simulink model "c00012M_harness"  (R2018a)
settings: Solver=FixedStepAuto  StartTime=0.0  StopTime=300  FixedStep=0.1  RelTol=1e-3
undefined symbols (not defined in the file): A1, hmax, PriorityTank, R1, R2, sigbuilder_block
(part 1 of 19)
settings Model: Creator=aarrieta  LastModifiedBy=umarkiegi

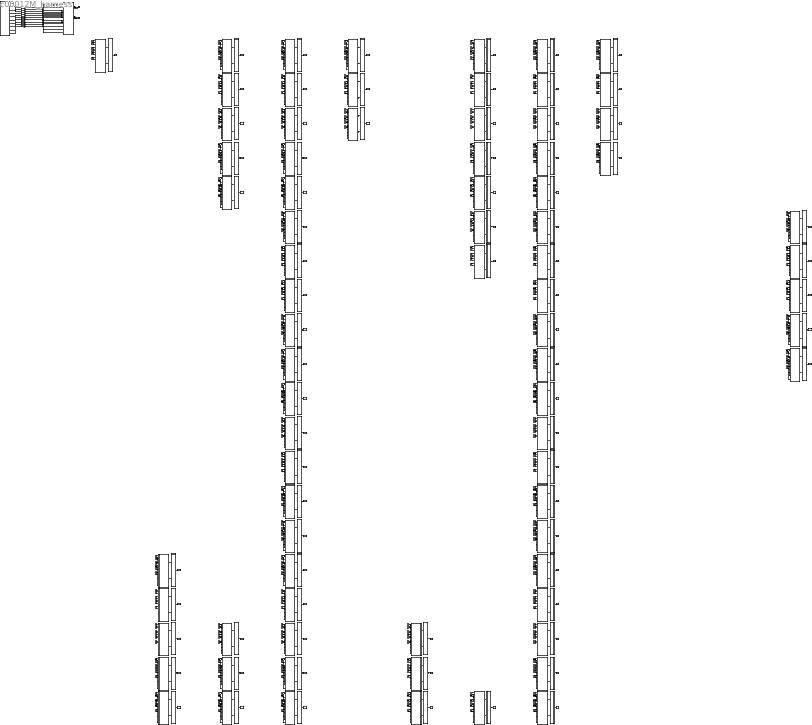
== system c00012M_harness ==
  CPSUT : Subsystem
  Eval : Subsystem
  Eval117 : Subsystem
  Eval118 : Subsystem
  Eval119 : Subsystem
  Eval120 : Subsystem
  Eval121 : Subsystem
  Eval122 : Subsystem
  Eval123 : Subsystem
  Eval124 : Subsystem
  Eval125 : Subsystem
  Eval126 : Subsystem
  Eval139 : Subsystem
  Eval140 : Subsystem
  Eval141 : Subsystem
  Eval142 : Subsystem
  Eval143 : Subsystem
  Eval144 : Subsystem
  Eval145 : Subsystem
  Eval146 : Subsystem
  Eval147 : Subsystem
  Eval148 : Subsystem
  Eval149 : Subsystem
  Eval150 : Subsystem
  Eval151 : Subsystem
  Eval152 : Subsystem
  Eval153 : Subsystem
  Eval154 : Subsystem
  Eval155 : Subsystem
  Eval156 : Subsystem
  Eval157 : Subsystem
  Eval158 : Subsystem
  Eval159 : Subsystem
  Eval160 : Subsystem
  Eval161 : Subsystem
  Eval162 : Subsystem
  Eval163 : Subsystem
  Eval225 : Subsystem
  Eval226 : Subsystem
  Eval227 : Subsystem
  Eval228 : Subsystem
  Eval229 : Subsystem
  Eval35 : Subsystem
  Eval36 : Subsystem
  Eval37 : Subsystem
  Eval38 : Subsystem
  Eval39 : Subsystem
  Eval40 : Subsystem
  Eval41 : Subsystem
  Eval42 : Subsystem
  Eval43 : Subsystem
  Eval44 : Subsystem
  Eval57 : Subsystem
  Eval58 : Subsystem
  Eval59 : Subsystem
  Eval60 : Subsystem
  Eval61 : Subsystem
  Eval62 : Subsystem
  Eval63 : Subsystem
  Eval64 : Subsystem
  Eval65 : Subsystem
  Eval66 : Subsystem
  Eval67 : Subsystem
  Eval68 : Subsystem
  Eval69 : Subsystem
  Eval70 : Subsystem
  Eval71 : Subsystem
  Eval72 : Subsystem
  Eval73 : Subsystem
  Eval74 : Subsystem
  Eval75 : Subsystem
  Eval76 : Subsystem
  Eval77 : Subsystem
  Eval78 : Subsystem
  Eval79 : Subsystem
  Eval80 : Subsystem
  Eval81 : Subsystem
  Eval82 : Subsystem
  Inputs : Subsystem  Tag=STV Subsys  LoadFcn=sigbuilder_block('load');  StartFcn=sigbuilder_block('start');  StopFcn=sigbuilder_block('stop');  ClipboardFcn=sigbuilder_block('clipboard');  mask(Sigbuilder block){tuvar=[0:10]}
      mask init:
      | if ~strcmp(get_param(bdroot(gcb),'SimulationStatus'),'stopped'),tuvar = sigbuilder_block('maskInit'); end
      settings: CopyFcn=sigbuilder_block('copy');  DeleteFcn=sigbuilder_block('delete');  ModelCloseFcn=sigbuilder_block('modelClose');  PreSaveFcn=sigbuilder_block('preSave');  PauseFcn=sigbuilder_block('pause');  ContinueFcn=sigbuilder_block('continue');  NameChangeFcn=sigbuilder_block('namechange');  OpenFcn=sigbuilder_block('open',[276.75 163.5 675.75 486.75 ]);  CloseFcn=sigbuilder_block('close');
      mask Display: plot(0, 0, 100, 100,[2, 2, 32, 32, 2], [68, 8, 8, 68, 68],[32, 2], [38, 38], [32, 19, 2],[53, 60, 44], [32, 17, 17, 2],[16, 16, 31, 31]);txt = getActiveGroup(gcbh);text(2, 100, txt,'verticalAlignment', 'top');
  M001 : Subsystem
  M036 : Subsystem
  M037 : Subsystem
  M038 : Subsystem
  M039 : Subsystem
  M040 : Subsystem
  M041 : Subsystem
  M042 : Subsystem
  M043 : Subsystem
  M044 : Subsystem
  M045 : Subsystem
  M058 : Subsystem
  M059 : Subsystem
  M060 : Subsystem
  M061 : Subsystem
  M062 : Subsystem
  M063 : Subsystem
  M064 : Subsystem
  M065 : Subsystem
  M066 : Subsystem
  M067 : Subsystem
  M068 : Subsystem
  M069 : Subsystem
  M070 : Subsystem
  M071 : Subsystem
  M072 : Subsystem
  M073 : Subsystem
  M074 : Subsystem
  M075 : Subsystem
  M076 : Subsystem
  M077 : Subsystem
  M078 : Subsystem
  M079 : Subsystem
  M080 : Subsystem
  M081 : Subsystem
  M082 : Subsystem
  M083 : Subsystem
  M118 : Subsystem
  M119 : Subsystem
  M120 : Subsystem
  M121 : Subsystem
  M122 : Subsystem
  M123 : Subsystem
  M124 : Subsystem
  M125 : Subsystem
  M126 : Subsystem
  M127 : Subsystem
  M140 : Subsystem
  M141 : Subsystem
  M142 : Subsystem
  M143 : Subsystem
  M144 : Subsystem
  M145 : Subsystem
  M146 : Subsystem
  M147 : Subsystem
  M148 : Subsystem
  M149 : Subsystem
  M150 : Subsystem
  M151 : Subsystem
  M152 : Subsystem
  M153 : Subsystem
  M154 : Subsystem
  M155 : Subsystem
  M156 : Subsystem
  M157 : Subsystem
  M158 : Subsystem
  M159 : Subsystem
  M160 : Subsystem
  M161 : Subsystem
  M162 : Subsystem
  M163 : Subsystem
  M164 : Subsystem
  M226 : Subsystem
  M227 : Subsystem
  M228 : Subsystem
  M229 : Subsystem
  M230 : Subsystem
  To Workspace : ToWorkspace  VariableName=mutant001  SampleTime=-1
  To Workspace117 : ToWorkspace  VariableName=mutant118  SampleTime=-1
  To Workspace118 : ToWorkspace  VariableName=mutant119  SampleTime=-1
  To Workspace119 : ToWorkspace  VariableName=mutant120  SampleTime=-1
  To Workspace120 : ToWorkspace  VariableName=mutant121  SampleTime=-1
  To Workspace121 : ToWorkspace  VariableName=mutant122  SampleTime=-1
  To Workspace122 : ToWorkspace  VariableName=mutant123  SampleTime=-1
  To Workspace123 : ToWorkspace  VariableName=mutant124  SampleTime=-1
  To Workspace124 : ToWorkspace  VariableName=mutant125  SampleTime=-1
  To Workspace125 : ToWorkspace  VariableName=mutant126  SampleTime=-1
  To Workspace126 : ToWorkspace  VariableName=mutant127  SampleTime=-1
  To Workspace139 : ToWorkspace  VariableName=mutant140  SampleTime=-1
  To Workspace140 : ToWorkspace  VariableName=mutant141  SampleTime=-1
  To Workspace141 : ToWorkspace  VariableName=mutant142  SampleTime=-1
  To Workspace142 : ToWorkspace  VariableName=mutant143  SampleTime=-1
  To Workspace143 : ToWorkspace  VariableName=mutant144  SampleTime=-1
  To Workspace144 : ToWorkspace  VariableName=mutant145  SampleTime=-1
  To Workspace145 : ToWorkspace  VariableName=mutant146  SampleTime=-1
  To Workspace146 : ToWorkspace  VariableName=mutant147  SampleTime=-1
  To Workspace147 : ToWorkspace  VariableName=mutant148  SampleTime=-1
  To Workspace148 : ToWorkspace  VariableName=mutant149  SampleTime=-1
  To Workspace149 : ToWorkspace  VariableName=mutant150  SampleTime=-1
  To Workspace150 : ToWorkspace  VariableName=mutant151  SampleTime=-1
  To Workspace151 : ToWorkspace  VariableName=mutant152  SampleTime=-1
  To Workspace152 : ToWorkspace  VariableName=mutant153  SampleTime=-1
  To Workspace153 : ToWorkspace  VariableName=mutant154  SampleTime=-1
  To Workspace154 : ToWorkspace  VariableName=mutant155  SampleTime=-1
  To Workspace155 : ToWorkspace  VariableName=mutant156  SampleTime=-1
  To Workspace156 : ToWorkspace  VariableName=mutant157  SampleTime=-1
  To Workspace157 : ToWorkspace  VariableName=mutant158  SampleTime=-1
  To Workspace158 : ToWorkspace  VariableName=mutant159  SampleTime=-1
  To Workspace159 : ToWorkspace  VariableName=mutant160  SampleTime=-1
  To Workspace160 : ToWorkspace  VariableName=mutant161  SampleTime=-1
  To Workspace161 : ToWorkspace  VariableName=mutant162  SampleTime=-1
  To Workspace162 : ToWorkspace  VariableName=mutant163  SampleTime=-1
  To Workspace163 : ToWorkspace  VariableName=mutant164  SampleTime=-1
  To Workspace225 : ToWorkspace  VariableName=mutant226  SampleTime=-1
  To Workspace226 : ToWorkspace  VariableName=mutant227  SampleTime=-1
  To Workspace227 : ToWorkspace  VariableName=mutant228  SampleTime=-1
  To Workspace228 : ToWorkspace  VariableName=mutant229  SampleTime=-1
  To Workspace229 : ToWorkspace  VariableName=mutant230  SampleTime=-1
  To Workspace35 : ToWorkspace  VariableName=mutant036  SampleTime=-1
  To Workspace36 : ToWorkspace  VariableName=mutant037  SampleTime=-1
  To Workspace37 : ToWorkspace  VariableName=mutant038  SampleTime=-1
  To Workspace38 : ToWorkspace  VariableName=mutant039  SampleTime=-1
  To Workspace39 : ToWorkspace  VariableName=mutant040  SampleTime=-1
  To Workspace40 : ToWorkspace  VariableName=mutant041  SampleTime=-1
  To Workspace41 : ToWorkspace  VariableName=mutant042  SampleTime=-1
  To Workspace42 : ToWorkspace  VariableName=mutant043  SampleTime=-1
  To Workspace43 : ToWorkspace  VariableName=mutant044  SampleTime=-1
  To Workspace44 : ToWorkspace  VariableName=mutant045  SampleTime=-1
  To Workspace57 : ToWorkspace  VariableName=mutant058  SampleTime=-1
  To Workspace58 : ToWorkspace  VariableName=mutant059  SampleTime=-1
  To Workspace59 : ToWorkspace  VariableName=mutant060  SampleTime=-1
  To Workspace60 : ToWorkspace  VariableName=mutant061  SampleTime=-1
  To Workspace61 : ToWorkspace  VariableName=mutant062  SampleTime=-1
  To Workspace62 : ToWorkspace  VariableName=mutant063  SampleTime=-1
  To Workspace63 : ToWorkspace  VariableName=mutant064  SampleTime=-1
  To Workspace64 : ToWorkspace  VariableName=mutant065  SampleTime=-1
  To Workspace65 : ToWorkspace  VariableName=mutant066  SampleTime=-1
  To Workspace66 : ToWorkspace  VariableName=mutant067  SampleTime=-1
  To Workspace67 : ToWorkspace  VariableName=mutant068  SampleTime=-1
  To Workspace68 : ToWorkspace  VariableName=mutant069  SampleTime=-1
  To Workspace69 : ToWorkspace  VariableName=mutant070  SampleTime=-1
  To Workspace70 : ToWorkspace  VariableName=mutant071  SampleTime=-1
  To Workspace71 : ToWorkspace  VariableName=mutant072  SampleTime=-1
  To Workspace72 : ToWorkspace  VariableName=mutant073  SampleTime=-1
  To Workspace73 : ToWorkspace  VariableName=mutant074  SampleTime=-1
  To Workspace74 : ToWorkspace  VariableName=mutant075  SampleTime=-1
  To Workspace75 : ToWorkspace  VariableName=mutant076  SampleTime=-1
  To Workspace76 : ToWorkspace  VariableName=mutant077  SampleTime=-1
  To Workspace77 : ToWorkspace  VariableName=mutant078  SampleTime=-1
  To Workspace78 : ToWorkspace  VariableName=mutant079  SampleTime=-1
  To Workspace79 : ToWorkspace  VariableName=mutant080  SampleTime=-1
  To Workspace80 : ToWorkspace  VariableName=mutant081  SampleTime=-1
  To Workspace81 : ToWorkspace  VariableName=mutant082  SampleTime=-1
  To Workspace82 : ToWorkspace  VariableName=mutant083  SampleTime=-1
  dtc_CT1 : DataTypeConversion
  dtc_CT2 : DataTypeConversion
  dtc_E1 : DataTypeConversion
  dtc_E2 : DataTypeConversion
  dtc_EB1 : DataTypeConversion
  dtc_EB2 : DataTypeConversion
  dtc_F1 : DataTypeConversion
  dtc_F2 : DataTypeConversion
  dtc_T1 : DataTypeConversion
  dtc_T2 : DataTypeConversion
  LL1 : Outport
  LL2 : Outport  Port=2
  tag scope: out1=global, out2=global
  wires:
  CPSUT/1(LL1) -> [out1], LL1/1
  CPSUT/2(LL2) -> [out2], LL2/1
  [in1] -> M001/1(CT1)
  [in2] -> M001/2(F1)
  [in3] -> M001/3(E1)
  [in5] -> M001/4(T1)
  [in6] -> M001/5(EB1)
  [in7] -> M001/6(CT2)
  [in8] -> M001/7(F2)
  [in9] -> M001/8(E2)
  [in11] -> M001/9(T2)
  [in12] -> M001/10(EB2)
  Eval/1(Out1) -> To Workspace/1
  M001/1(LL1) -> Eval/1(In1)
  M001/2(LL2) -> Eval/2(In2)
  [in1] -> M036/1(CT1)
  [in2] -> M036/2(F1)
  [in3] -> M036/3(E1)
  [in5] -> M036/4(T1)
  [in6] -> M036/5(EB1)
  [in7] -> M036/6(CT2)
  [in8] -> M036/7(F2)
  [in9] -> M036/8(E2)
  [in11] -> M036/9(T2)
  [in12] -> M036/10(EB2)
  M036/1(LL1) -> Eval35/1(In1)
  M036/2(LL2) -> Eval35/2(In2)
  Eval35/1(Out1) -> To Workspace35/1
  [in1] -> M037/1(CT1)
  [in2] -> M037/2(F1)
  [in3] -> M037/3(E1)
  [in5] -> M037/4(T1)
  [in6] -> M037/5(EB1)
  [in7] -> M037/6(CT2)
  [in8] -> M037/7(F2)
  [in9] -> M037/8(E2)
  [in11] -> M037/9(T2)
  [in12] -> M037/10(EB2)
  M037/1(LL1) -> Eval36/1(In1)
  M037/2(LL2) -> Eval36/2(In2)
  Eval36/1(Out1) -> To Workspace36/1
  [in1] -> M038/1(CT1)
  [in2] -> M038/2(F1)
  [in3] -> M038/3(E1)
  [in5] -> M038/4(T1)
  [in6] -> M038/5(EB1)
  [in7] -> M038/6(CT2)
  [in8] -> M038/7(F2)
  [in9] -> M038/8(E2)
  [in11] -> M038/9(T2)
  [in12] -> M038/10(EB2)
  M038/1(LL1) -> Eval37/1(In1)
  M038/2(LL2) -> Eval37/2(In2)
  Eval37/1(Out1) -> To Workspace37/1
  [in1] -> M039/1(CT1)
  [in2] -> M039/2(F1)
  [in3] -> M039/3(E1)
  [in5] -> M039/4(T1)
  [in6] -> M039/5(EB1)
  [in7] -> M039/6(CT2)
  [in8] -> M039/7(F2)
  [in9] -> M039/8(E2)
  [in11] -> M039/9(T2)
  [in12] -> M039/10(EB2)
  M039/1(LL1) -> Eval38/1(In1)
  M039/2(LL2) -> Eval38/2(In2)
  Eval38/1(Out1) -> To Workspace38/1
  [in1] -> M040/1(CT1)
  [in2] -> M040/2(F1)
  [in3] -> M040/3(E1)
  [in5] -> M040/4(T1)
  [in6] -> M040/5(EB1)
  [in7] -> M040/6(CT2)
  [in8] -> M040/7(F2)
  [in9] -> M040/8(E2)
  [in11] -> M040/9(T2)
  [in12] -> M040/10(EB2)
  M040/1(LL1) -> Eval39/1(In1)
  M040/2(LL2) -> Eval39/2(In2)
  Eval39/1(Out1) -> To Workspace39/1
  [in1] -> M041/1(CT1)
  [in2] -> M041/2(F1)
  [in3] -> M041/3(E1)
  [in5] -> M041/4(T1)
  [in6] -> M041/5(EB1)
  [in7] -> M041/6(CT2)
  [in8] -> M041/7(F2)
  [in9] -> M041/8(E2)
  [in11] -> M041/9(T2)
  [in12] -> M041/10(EB2)
  M041/1(LL1) -> Eval40/1(In1)
  M041/2(LL2) -> Eval40/2(In2)
  Eval40/1(Out1) -> To Workspace40/1
  [in1] -> M042/1(CT1)
  [in2] -> M042/2(F1)
  [in3] -> M042/3(E1)
  [in5] -> M042/4(T1)
  [in6] -> M042/5(EB1)
  [in7] -> M042/6(CT2)
  [in8] -> M042/7(F2)
  [in9] -> M042/8(E2)
  [in11] -> M042/9(T2)
  [in12] -> M042/10(EB2)
  M042/1(LL1) -> Eval41/1(In1)
  M042/2(LL2) -> Eval41/2(In2)
  Eval41/1(Out1) -> To Workspace41/1
  [in1] -> M043/1(CT1)
  [in2] -> M043/2(F1)
  [in3] -> M043/3(E1)
  [in5] -> M043/4(T1)
  [in6] -> M043/5(EB1)
  [in7] -> M043/6(CT2)
  [in8] -> M043/7(F2)
  [in9] -> M043/8(E2)
  [in11] -> M043/9(T2)
  [in12] -> M043/10(EB2)
  M043/1(LL1) -> Eval42/1(In1)
  M043/2(LL2) -> Eval42/2(In2)
  Eval42/1(Out1) -> To Workspace42/1
  [in1] -> M044/1(CT1)
  [in2] -> M044/2(F1)
  [in3] -> M044/3(E1)
  [in5] -> M044/4(T1)
  [in6] -> M044/5(EB1)
  [in7] -> M044/6(CT2)
  [in8] -> M044/7(F2)
  [in9] -> M044/8(E2)
  [in11] -> M044/9(T2)
  [in12] -> M044/10(EB2)
  M044/1(LL1) -> Eval43/1(In1)
  M044/2(LL2) -> Eval43/2(In2)
  Eval43/1(Out1) -> To Workspace43/1
  [in1] -> M045/1(CT1)
  [in2] -> M045/2(F1)
  [in3] -> M045/3(E1)
  [in5] -> M045/4(T1)
  [in6] -> M045/5(EB1)
  [in7] -> M045/6(CT2)
  [in8] -> M045/7(F2)
  [in9] -> M045/8(E2)
  [in11] -> M045/9(T2)
  [in12] -> M045/10(EB2)
  M045/1(LL1) -> Eval44/1(In1)
  M045/2(LL2) -> Eval44/2(In2)
  Eval44/1(Out1) -> To Workspace44/1
  [in1] -> M058/1(CT1)
  [in2] -> M058/2(F1)
  [in3] -> M058/3(E1)
  [in5] -> M058/4(T1)
  [in6] -> M058/5(EB1)
  [in7] -> M058/6(CT2)
  [in8] -> M058/7(F2)
  [in9] -> M058/8(E2)
  [in11] -> M058/9(T2)
  [in12] -> M058/10(EB2)
  M058/1(LL1) -> Eval57/1(In1)
  M058/2(LL2) -> Eval57/2(In2)
  Eval57/1(Out1) -> To Workspace57/1
  [in1] -> M059/1(CT1)
  [in2] -> M059/2(F1)
  [in3] -> M059/3(E1)
  [in5] -> M059/4(T1)
  [in6] -> M059/5(EB1)
  [in7] -> M059/6(CT2)
  [in8] -> M059/7(F2)
  [in9] -> M059/8(E2)
  [in11] -> M059/9(T2)
  [in12] -> M059/10(EB2)
  M059/1(LL1) -> Eval58/1(In1)
  M059/2(LL2) -> Eval58/2(In2)
  Eval58/1(Out1) -> To Workspace58/1
  [in1] -> M060/1(CT1)
  [in2] -> M060/2(F1)
  [in3] -> M060/3(E1)
  [in5] -> M060/4(T1)
  [in6] -> M060/5(EB1)
  [in7] -> M060/6(CT2)
  [in8] -> M060/7(F2)
  [in9] -> M060/8(E2)
  [in11] -> M060/9(T2)
  [in12] -> M060/10(EB2)
  M060/1(LL1) -> Eval59/1(In1)
  M060/2(LL2) -> Eval59/2(In2)
  Eval59/1(Out1) -> To Workspace59/1
  [in1] -> M061/1(CT1)
  [in2] -> M061/2(F1)
  [in3] -> M061/3(E1)
  [in5] -> M061/4(T1)
  [in6] -> M061/5(EB1)
  [in7] -> M061/6(CT2)
  [in8] -> M061/7(F2)
  [in9] -> M061/8(E2)
  [in11] -> M061/9(T2)
  [in12] -> M061/10(EB2)
  M061/1(LL1) -> Eval60/1(In1)
  M061/2(LL2) -> Eval60/2(In2)
  Eval60/1(Out1) -> To Workspace60/1
  [in1] -> M062/1(CT1)
  [in2] -> M062/2(F1)
  [in3] -> M062/3(E1)
  [in5] -> M062/4(T1)
  [in6] -> M062/5(EB1)
  [in7] -> M062/6(CT2)
  [in8] -> M062/7(F2)
  [in9] -> M062/8(E2)
  [in11] -> M062/9(T2)
  [in12] -> M062/10(EB2)
  M062/1(LL1) -> Eval61/1(In1)
  M062/2(LL2) -> Eval61/2(In2)
  Eval61/1(Out1) -> To Workspace61/1
  [in1] -> M063/1(CT1)
  [in2] -> M063/2(F1)
  [in3] -> M063/3(E1)
  [in5] -> M063/4(T1)
  [in6] -> M063/5(EB1)
  [in7] -> M063/6(CT2)
  [in8] -> M063/7(F2)
  [in9] -> M063/8(E2)
  [in11] -> M063/9(T2)
  [in12] -> M063/10(EB2)
  M063/1(LL1) -> Eval62/1(In1)
  M063/2(LL2) -> Eval62/2(In2)
  Eval62/1(Out1) -> To Workspace62/1
  [in1] -> M064/1(CT1)
  [in2] -> M064/2(F1)
  [in3] -> M064/3(E1)
  [in5] -> M064/4(T1)
  [in6] -> M064/5(EB1)
  [in7] -> M064/6(CT2)
  [in8] -> M064/7(F2)
  [in9] -> M064/8(E2)
  [in11] -> M064/9(T2)
  [in12] -> M064/10(EB2)
  M064/1(LL1) -> Eval63/1(In1)
  M064/2(LL2) -> Eval63/2(In2)
  Eval63/1(Out1) -> To Workspace63/1
  [in1] -> M065/1(CT1)
  [in2] -> M065/2(F1)
  [in3] -> M065/3(E1)
  [in5] -> M065/4(T1)
  [in6] -> M065/5(EB1)
  [in7] -> M065/6(CT2)
  [in8] -> M065/7(F2)
  [in9] -> M065/8(E2)
  [in11] -> M065/9(T2)
  [in12] -> M065/10(EB2)
  M065/1(LL1) -> Eval64/1(In1)
  M065/2(LL2) -> Eval64/2(In2)
  Eval64/1(Out1) -> To Workspace64/1
  [in1] -> M066/1(CT1)
  [in2] -> M066/2(F1)
  [in3] -> M066/3(E1)
  [in5] -> M066/4(T1)
  [in6] -> M066/5(EB1)
  [in7] -> M066/6(CT2)
  [in8] -> M066/7(F2)
  [in9] -> M066/8(E2)
  [in11] -> M066/9(T2)
  [in12] -> M066/10(EB2)
  M066/1(LL1) -> Eval65/1(In1)
  M066/2(LL2) -> Eval65/2(In2)
  Eval65/1(Out1) -> To Workspace65/1
  [in1] -> M067/1(CT1)
  [in2] -> M067/2(F1)
  [in3] -> M067/3(E1)
  [in5] -> M067/4(T1)
  [in6] -> M067/5(EB1)
  [in7] -> M067/6(CT2)
  [in8] -> M067/7(F2)
  [in9] -> M067/8(E2)
  [in11] -> M067/9(T2)
  [in12] -> M067/10(EB2)
  M067/1(LL1) -> Eval66/1(In1)
  M067/2(LL2) -> Eval66/2(In2)
  Eval66/1(Out1) -> To Workspace66/1
  [in1] -> M068/1(CT1)
  [in2] -> M068/2(F1)
  [in3] -> M068/3(E1)
  [in5] -> M068/4(T1)
  [in6] -> M068/5(EB1)
  [in7] -> M068/6(CT2)
  [in8] -> M068/7(F2)
  [in9] -> M068/8(E2)
  [in11] -> M068/9(T2)
  [in12] -> M068/10(EB2)
  M068/1(LL1) -> Eval67/1(In1)
  M068/2(LL2) -> Eval67/2(In2)
  Eval67/1(Out1) -> To Workspace67/1
  [in1] -> M069/1(CT1)
  [in2] -> M069/2(F1)
  [in3] -> M069/3(E1)
  [in5] -> M069/4(T1)
  [in6] -> M069/5(EB1)
  [in7] -> M069/6(CT2)
  [in8] -> M069/7(F2)
  [in9] -> M069/8(E2)
  [in11] -> M069/9(T2)
  [in12] -> M069/10(EB2)
  M069/1(LL1) -> Eval68/1(In1)
  M069/2(LL2) -> Eval68/2(In2)
  Eval68/1(Out1) -> To Workspace68/1
  [in1] -> M070/1(CT1)
  [in2] -> M070/2(F1)
  [in3] -> M070/3(E1)
  [in5] -> M070/4(T1)
  [in6] -> M070/5(EB1)
  [in7] -> M070/6(CT2)
  [in8] -> M070/7(F2)
  [in9] -> M070/8(E2)
  [in11] -> M070/9(T2)
  [in12] -> M070/10(EB2)
  M070/1(LL1) -> Eval69/1(In1)
  M070/2(LL2) -> Eval69/2(In2)
  Eval69/1(Out1) -> To Workspace69/1
  [in1] -> M071/1(CT1)
  [in2] -> M071/2(F1)
  [in3] -> M071/3(E1)
  [in5] -> M071/4(T1)
  [in6] -> M071/5(EB1)
  [in7] -> M071/6(CT2)
  [in8] -> M071/7(F2)
  [in9] -> M071/8(E2)
  [in11] -> M071/9(T2)
  [in12] -> M071/10(EB2)
  M071/1(LL1) -> Eval70/1(In1)
  M071/2(LL2) -> Eval70/2(In2)
  Eval70/1(Out1) -> To Workspace70/1
  [in1] -> M072/1(CT1)
  [in2] -> M072/2(F1)
  [in3] -> M072/3(E1)
  [in5] -> M072/4(T1)
  [in6] -> M072/5(EB1)
  [in7] -> M072/6(CT2)
  [in8] -> M072/7(F2)
  [in9] -> M072/8(E2)
  [in11] -> M072/9(T2)
  [in12] -> M072/10(EB2)
  M072/1(LL1) -> Eval71/1(In1)
  M072/2(LL2) -> Eval71/2(In2)
  Eval71/1(Out1) -> To Workspace71/1
  [in1] -> M073/1(CT1)
  [in2] -> M073/2(F1)
  [in3] -> M073/3(E1)
  [in5] -> M073/4(T1)
  [in6] -> M073/5(EB1)
  [in7] -> M073/6(CT2)
  [in8] -> M073/7(F2)
  [in9] -> M073/8(E2)
  [in11] -> M073/9(T2)
  [in12] -> M073/10(EB2)
  M073/1(LL1) -> Eval72/1(In1)
  M073/2(LL2) -> Eval72/2(In2)
  Eval72/1(Out1) -> To Workspace72/1
  [in1] -> M074/1(CT1)
  [in2] -> M074/2(F1)
  [in3] -> M074/3(E1)
  [in5] -> M074/4(T1)
  [in6] -> M074/5(EB1)
  [in7] -> M074/6(CT2)
  [in8] -> M074/7(F2)
  [in9] -> M074/8(E2)
  [in11] -> M074/9(T2)
  [in12] -> M074/10(EB2)
  M074/1(LL1) -> Eval73/1(In1)
  M074/2(LL2) -> Eval73/2(In2)
  Eval73/1(Out1) -> To Workspace73/1
  [in1] -> M075/1(CT1)
  [in2] -> M075/2(F1)
  [in3] -> M075/3(E1)
  [in5] -> M075/4(T1)
  [in6] -> M075/5(EB1)
  [in7] -> M075/6(CT2)
  [in8] -> M075/7(F2)
  [in9] -> M075/8(E2)
  [in11] -> M075/9(T2)
  [in12] -> M075/10(EB2)
  M075/1(LL1) -> Eval74/1(In1)
  M075/2(LL2) -> Eval74/2(In2)
  Eval74/1(Out1) -> To Workspace74/1
  [in1] -> M076/1(CT1)
  [in2] -> M076/2(F1)
  [in3] -> M076/3(E1)
  [in5] -> M076/4(T1)
  [in6] -> M076/5(EB1)
  [in7] -> M076/6(CT2)
  [in8] -> M076/7(F2)
  [in9] -> M076/8(E2)
  [in11] -> M076/9(T2)
  [in12] -> M076/10(EB2)
  M076/1(LL1) -> Eval75/1(In1)
  M076/2(LL2) -> Eval75/2(In2)
  Eval75/1(Out1) -> To Workspace75/1
  [in1] -> M077/1(CT1)
  [in2] -> M077/2(F1)
  [in3] -> M077/3(E1)
  [in5] -> M077/4(T1)
  [in6] -> M077/5(EB1)
  [in7] -> M077/6(CT2)
  [in8] -> M077/7(F2)
  [in9] -> M077/8(E2)
  [in11] -> M077/9(T2)
  [in12] -> M077/10(EB2)
  M077/1(LL1) -> Eval76/1(In1)
  M077/2(LL2) -> Eval76/2(In2)
  Eval76/1(Out1) -> To Workspace76/1
  [in1] -> M078/1(CT1)
  [in2] -> M078/2(F1)
  [in3] -> M078/3(E1)
  [in5] -> M078/4(T1)
  [in6] -> M078/5(EB1)
  [in7] -> M078/6(CT2)
  [in8] -> M078/7(F2)
  [in9] -> M078/8(E2)
  [in11] -> M078/9(T2)
  [in12] -> M078/10(EB2)
  M078/1(LL1) -> Eval77/1(In1)
  M078/2(LL2) -> Eval77/2(In2)
  Eval77/1(Out1) -> To Workspace77/1
  [in1] -> M079/1(CT1)
  [in2] -> M079/2(F1)
  [in3] -> M079/3(E1)
  [in5] -> M079/4(T1)
  [in6] -> M079/5(EB1)
  [in7] -> M079/6(CT2)
  [in8] -> M079/7(F2)
  [in9] -> M079/8(E2)
  [in11] -> M079/9(T2)
  [in12] -> M079/10(EB2)
  M079/1(LL1) -> Eval78/1(In1)
  M079/2(LL2) -> Eval78/2(In2)
  Eval78/1(Out1) -> To Workspace78/1
  [in1] -> M080/1(CT1)
  [in2] -> M080/2(F1)
  [in3] -> M080/3(E1)
  [in5] -> M080/4(T1)
  [in6] -> M080/5(EB1)
  [in7] -> M080/6(CT2)
  [in8] -> M080/7(F2)
  [in9] -> M080/8(E2)
  [in11] -> M080/9(T2)
  [in12] -> M080/10(EB2)
  M080/1(LL1) -> Eval79/1(In1)
  M080/2(LL2) -> Eval79/2(In2)
  Eval79/1(Out1) -> To Workspace79/1
  [in1] -> M081/1(CT1)
  [in2] -> M081/2(F1)
  [in3] -> M081/3(E1)
  [in5] -> M081/4(T1)
  [in6] -> M081/5(EB1)
  [in7] -> M081/6(CT2)
  [in8] -> M081/7(F2)
  [in9] -> M081/8(E2)
  [in11] -> M081/9(T2)
  [in12] -> M081/10(EB2)
  M081/1(LL1) -> Eval80/1(In1)
  M081/2(LL2) -> Eval80/2(In2)
  Eval80/1(Out1) -> To Workspace80/1
  [in1] -> M082/1(CT1)
  [in2] -> M082/2(F1)
  [in3] -> M082/3(E1)
  [in5] -> M082/4(T1)
  [in6] -> M082/5(EB1)
  [in7] -> M082/6(CT2)
  [in8] -> M082/7(F2)
  [in9] -> M082/8(E2)
  [in11] -> M082/9(T2)
  [in12] -> M082/10(EB2)
  M082/1(LL1) -> Eval81/1(In1)
  M082/2(LL2) -> Eval81/2(In2)
  Eval81/1(Out1) -> To Workspace81/1
  [in1] -> M083/1(CT1)
  [in2] -> M083/2(F1)
  [in3] -> M083/3(E1)
  [in5] -> M083/4(T1)
  [in6] -> M083/5(EB1)
  [in7] -> M083/6(CT2)
  [in8] -> M083/7(F2)
  [in9] -> M083/8(E2)
  [in11] -> M083/9(T2)
  [in12] -> M083/10(EB2)
  M083/1(LL1) -> Eval82/1(In1)
  M083/2(LL2) -> Eval82/2(In2)
  Eval82/1(Out1) -> To Workspace82/1
  [in1] -> M118/1(CT1)
  [in2] -> M118/2(F1)
  [in3] -> M118/3(E1)
  [in5] -> M118/4(T1)
  [in6] -> M118/5(EB1)
  [in7] -> M118/6(CT2)
  [in8] -> M118/7(F2)
  [in9] -> M118/8(E2)
  [in11] -> M118/9(T2)
  [in12] -> M118/10(EB2)
  M118/1(LL1) -> Eval117/1(In1)
  M118/2(LL2) -> Eval117/2(In2)
  Eval117/1(Out1) -> To Workspace117/1
  [in1] -> M119/1(CT1)
  [in2] -> M119/2(F1)
  [in3] -> M119/3(E1)
  [in5] -> M119/4(T1)
  [in6] -> M119/5(EB1)
  [in7] -> M119/6(CT2)
  [in8] -> M119/7(F2)
  [in9] -> M119/8(E2)
  [in11] -> M119/9(T2)
  [in12] -> M119/10(EB2)
  M119/1(LL1) -> Eval118/1(In1)
  M119/2(LL2) -> Eval118/2(In2)
  Eval118/1(Out1) -> To Workspace118/1
  [in1] -> M120/1(CT1)
  [in2] -> M120/2(F1)
  [in3] -> M120/3(E1)
  [in5] -> M120/4(T1)
  [in6] -> M120/5(EB1)
  [in7] -> M120/6(CT2)
  [in8] -> M120/7(F2)
  [in9] -> M120/8(E2)
  [in11] -> M120/9(T2)
  [in12] -> M120/10(EB2)
  M120/1(LL1) -> Eval119/1(In1)
  M120/2(LL2) -> Eval119/2(In2)
  Eval119/1(Out1) -> To Workspace119/1
  [in1] -> M121/1(CT1)
  [in2] -> M121/2(F1)
  [in3] -> M121/3(E1)
  [in5] -> M121/4(T1)
  [in6] -> M121/5(EB1)
  [in7] -> M121/6(CT2)
  [in8] -> M121/7(F2)
  [in9] -> M121/8(E2)
  [in11] -> M121/9(T2)
  [in12] -> M121/10(EB2)
  M121/1(LL1) -> Eval120/1(In1)
  M121/2(LL2) -> Eval120/2(In2)
  Eval120/1(Out1) -> To Workspace120/1
  [in1] -> M122/1(CT1)
  [in2] -> M122/2(F1)
  [in3] -> M122/3(E1)
  [in5] -> M122/4(T1)
  [in6] -> M122/5(EB1)
  [in7] -> M122/6(CT2)
  [in8] -> M122/7(F2)
  [in9] -> M122/8(E2)
  [in11] -> M122/9(T2)
  [in12] -> M122/10(EB2)
  M122/1(LL1) -> Eval121/1(In1)
  M122/2(LL2) -> Eval121/2(In2)
  Eval121/1(Out1) -> To Workspace121/1
  [in1] -> M123/1(CT1)
  [in2] -> M123/2(F1)
  [in3] -> M123/3(E1)
  [in5] -> M123/4(T1)
  [in6] -> M123/5(EB1)
  [in7] -> M123/6(CT2)
  [in8] -> M123/7(F2)
  [in9] -> M123/8(E2)
  [in11] -> M123/9(T2)
  [in12] -> M123/10(EB2)
  M123/1(LL1) -> Eval122/1(In1)
  M123/2(LL2) -> Eval122/2(In2)
  Eval122/1(Out1) -> To Workspace122/1
  [in1] -> M124/1(CT1)
  [in2] -> M124/2(F1)
  [in3] -> M124/3(E1)
  [in5] -> M124/4(T1)
  [in6] -> M124/5(EB1)
  [in7] -> M124/6(CT2)
  [in8] -> M124/7(F2)
  [in9] -> M124/8(E2)
  [in11] -> M124/9(T2)
  [in12] -> M124/10(EB2)
  M124/1(LL1) -> Eval123/1(In1)
  M124/2(LL2) -> Eval123/2(In2)
  Eval123/1(Out1) -> To Workspace123/1
  [in1] -> M125/1(CT1)
  [in2] -> M125/2(F1)
  [in3] -> M125/3(E1)
  [in5] -> M125/4(T1)
  [in6] -> M125/5(EB1)
  [in7] -> M125/6(CT2)
  [in8] -> M125/7(F2)
  [in9] -> M125/8(E2)
  [in11] -> M125/9(T2)
  [in12] -> M125/10(EB2)
  M125/1(LL1) -> Eval124/1(In1)
  M125/2(LL2) -> Eval124/2(In2)
  Eval124/1(Out1) -> To Workspace124/1
  [in1] -> M126/1(CT1)
  [in2] -> M126/2(F1)
  [in3] -> M126/3(E1)
  [in5] -> M126/4(T1)
  [in6] -> M126/5(EB1)
  [in7] -> M126/6(CT2)
  [in8] -> M126/7(F2)
  [in9] -> M126/8(E2)
  [in11] -> M126/9(T2)
  [in12] -> M126/10(EB2)
  M126/1(LL1) -> Eval125/1(In1)
  M126/2(LL2) -> Eval125/2(In2)
  Eval125/1(Out1) -> To Workspace125/1
  [in1] -> M127/1(CT1)
  [in2] -> M127/2(F1)
  [in3] -> M127/3(E1)
  [in5] -> M127/4(T1)
  [in6] -> M127/5(EB1)
  [in7] -> M127/6(CT2)
  [in8] -> M127/7(F2)
  [in9] -> M127/8(E2)
  [in11] -> M127/9(T2)
  [in12] -> M127/10(EB2)
  M127/1(LL1) -> Eval126/1(In1)
  M127/2(LL2) -> Eval126/2(In2)
  Eval126/1(Out1) -> To Workspace126/1
  [in1] -> M140/1(CT1)
  [in2] -> M140/2(F1)
  [in3] -> M140/3(E1)
  [in5] -> M140/4(T1)
  [in6] -> M140/5(EB1)
  [in7] -> M140/6(CT2)
  [in8] -> M140/7(F2)
  [in9] -> M140/8(E2)
  [in11] -> M140/9(T2)
  [in12] -> M140/10(EB2)
  M140/1(LL1) -> Eval139/1(In1)
  M140/2(LL2) -> Eval139/2(In2)
  Eval139/1(Out1) -> To Workspace139/1
  [in1] -> M141/1(CT1)
  [in2] -> M141/2(F1)
  [in3] -> M141/3(E1)
  [in5] -> M141/4(T1)
  [in6] -> M141/5(EB1)
  [in7] -> M141/6(CT2)
  [in8] -> M141/7(F2)
  [in9] -> M141/8(E2)
  [in11] -> M141/9(T2)
  [in12] -> M141/10(EB2)
  M141/1(LL1) -> Eval140/1(In1)
  M141/2(LL2) -> Eval140/2(In2)
  Eval140/1(Out1) -> To Workspace140/1
  [in1] -> M142/1(CT1)
  [in2] -> M142/2(F1)
  [in3] -> M142/3(E1)
  [in5] -> M142/4(T1)
  [in6] -> M142/5(EB1)
  [in7] -> M142/6(CT2)
  [in8] -> M142/7(F2)
  [in9] -> M142/8(E2)
  [in11] -> M142/9(T2)
  [in12] -> M142/10(EB2)
  M142/1(LL1) -> Eval141/1(In1)
  M142/2(LL2) -> Eval141/2(In2)
  Eval141/1(Out1) -> To Workspace141/1
  [in1] -> M143/1(CT1)
  [in2] -> M143/2(F1)
  [in3] -> M143/3(E1)
  [in5] -> M143/4(T1)
  [in6] -> M143/5(EB1)
  [in7] -> M143/6(CT2)
  [in8] -> M143/7(F2)
  [in9] -> M143/8(E2)
  [in11] -> M143/9(T2)
  [in12] -> M143/10(EB2)
  M143/1(LL1) -> Eval142/1(In1)
  M143/2(LL2) -> Eval142/2(In2)
  Eval142/1(Out1) -> To Workspace142/1
  [in1] -> M144/1(CT1)
  [in2] -> M144/2(F1)
  [in3] -> M144/3(E1)
  [in5] -> M144/4(T1)
  [in6] -> M144/5(EB1)
  [in7] -> M144/6(CT2)
  [in8] -> M144/7(F2)
  [in9] -> M144/8(E2)
  [in11] -> M144/9(T2)
  [in12] -> M144/10(EB2)
  M144/1(LL1) -> Eval143/1(In1)
  M144/2(LL2) -> Eval143/2(In2)
  Eval143/1(Out1) -> To Workspace143/1
  [in1] -> M145/1(CT1)
  [in2] -> M145/2(F1)
  [in3] -> M145/3(E1)
  [in5] -> M145/4(T1)
  [in6] -> M145/5(EB1)
  [in7] -> M145/6(CT2)
  [in8] -> M145/7(F2)
  [in9] -> M145/8(E2)
  [in11] -> M145/9(T2)
  [in12] -> M145/10(EB2)
  M145/1(LL1) -> Eval144/1(In1)
  M145/2(LL2) -> Eval144/2(In2)
  Eval144/1(Out1) -> To Workspace144/1
  [in1] -> M146/1(CT1)
  [in2] -> M146/2(F1)
  [in3] -> M146/3(E1)
  [in5] -> M146/4(T1)
  [in6] -> M146/5(EB1)
  [in7] -> M146/6(CT2)
  [in8] -> M146/7(F2)
  [in9] -> M146/8(E2)
  [in11] -> M146/9(T2)
  [in12] -> M146/10(EB2)
  M146/1(LL1) -> Eval145/1(In1)
  M146/2(LL2) -> Eval145/2(In2)
  Eval145/1(Out1) -> To Workspace145/1
  [in1] -> M147/1(CT1)
  [in2] -> M147/2(F1)
  [in3] -> M147/3(E1)
  [in5] -> M147/4(T1)
  [in6] -> M147/5(EB1)
  [in7] -> M147/6(CT2)
  [in8] -> M147/7(F2)
  [in9] -> M147/8(E2)
  [in11] -> M147/9(T2)
  [in12] -> M147/10(EB2)
  M147/1(LL1) -> Eval146/1(In1)
  M147/2(LL2) -> Eval146/2(In2)
  Eval146/1(Out1) -> To Workspace146/1
  [in1] -> M148/1(CT1)
  [in2] -> M148/2(F1)
  [in3] -> M148/3(E1)
  [in5] -> M148/4(T1)
  [in6] -> M148/5(EB1)
  [in7] -> M148/6(CT2)
  [in8] -> M148/7(F2)
  [in9] -> M148/8(E2)
  [in11] -> M148/9(T2)
  [in12] -> M148/10(EB2)
  M148/1(LL1) -> Eval147/1(In1)
  M148/2(LL2) -> Eval147/2(In2)
  Eval147/1(Out1) -> To Workspace147/1
  [in1] -> M149/1(CT1)
  [in2] -> M149/2(F1)
  [in3] -> M149/3(E1)
  [in5] -> M149/4(T1)
  [in6] -> M149/5(EB1)
  [in7] -> M149/6(CT2)
  [in8] -> M149/7(F2)
  [in9] -> M149/8(E2)
  [in11] -> M149/9(T2)
  [in12] -> M149/10(EB2)
  M149/1(LL1) -> Eval148/1(In1)
  M149/2(LL2) -> Eval148/2(In2)
  Eval148/1(Out1) -> To Workspace148/1
  [in1] -> M150/1(CT1)
  [in2] -> M150/2(F1)
  [in3] -> M150/3(E1)
  [in5] -> M150/4(T1)
  [in6] -> M150/5(EB1)
  [in7] -> M150/6(CT2)
  [in8] -> M150/7(F2)
  [in9] -> M150/8(E2)
  [in11] -> M150/9(T2)
  [in12] -> M150/10(EB2)
  M150/1(LL1) -> Eval149/1(In1)
  M150/2(LL2) -> Eval149/2(In2)
  Eval149/1(Out1) -> To Workspace149/1
  [in1] -> M151/1(CT1)
  [in2] -> M151/2(F1)
  [in3] -> M151/3(E1)
  [in5] -> M151/4(T1)
  [in6] -> M151/5(EB1)
  [in7] -> M151/6(CT2)
  [in8] -> M151/7(F2)
  [in9] -> M151/8(E2)
  [in11] -> M151/9(T2)
  [in12] -> M151/10(EB2)
  M151/1(LL1) -> Eval150/1(In1)
  M151/2(LL2) -> Eval150/2(In2)
  Eval150/1(Out1) -> To Workspace150/1
  [in1] -> M152/1(CT1)
  [in2] -> M152/2(F1)
  [in3] -> M152/3(E1)
  [in5] -> M152/4(T1)
  [in6] -> M152/5(EB1)
  [in7] -> M152/6(CT2)
  [in8] -> M152/7(F2)
  [in9] -> M152/8(E2)
  [in11] -> M152/9(T2)
  [in12] -> M152/10(EB2)
  M152/1(LL1) -> Eval151/1(In1)
  M152/2(LL2) -> Eval151/2(In2)
  Eval151/1(Out1) -> To Workspace151/1
  [in1] -> M153/1(CT1)
  [in2] -> M153/2(F1)
  [in3] -> M153/3(E1)
  [in5] -> M153/4(T1)
  [in6] -> M153/5(EB1)
  [in7] -> M153/6(CT2)
  [in8] -> M153/7(F2)
  [in9] -> M153/8(E2)
  [in11] -> M153/9(T2)
  [in12] -> M153/10(EB2)
  M153/1(LL1) -> Eval152/1(In1)
  M153/2(LL2) -> Eval152/2(In2)
  Eval152/1(Out1) -> To Workspace152/1
  [in1] -> M154/1(CT1)
  [in2] -> M154/2(F1)
  [in3] -> M154/3(E1)
  [in5] -> M154/4(T1)
  [in6] -> M154/5(EB1)
  [in7] -> M154/6(CT2)
  [in8] -> M154/7(F2)
  [in9] -> M154/8(E2)
  [in11] -> M154/9(T2)
  [in12] -> M154/10(EB2)
  M154/1(LL1) -> Eval153/1(In1)
  M154/2(LL2) -> Eval153/2(In2)
  Eval153/1(Out1) -> To Workspace153/1
  [in1] -> M155/1(CT1)
  [in2] -> M155/2(F1)
  [in3] -> M155/3(E1)
  [in5] -> M155/4(T1)
  [in6] -> M155/5(EB1)
  [in7] -> M155/6(CT2)
  [in8] -> M155/7(F2)
  [in9] -> M155/8(E2)
  [in11] -> M155/9(T2)
  [in12] -> M155/10(EB2)
  M155/1(LL1) -> Eval154/1(In1)
  M155/2(LL2) -> Eval154/2(In2)
  Eval154/1(Out1) -> To Workspace154/1
  [in1] -> M156/1(CT1)
  [in2] -> M156/2(F1)
  [in3] -> M156/3(E1)
  [in5] -> M156/4(T1)
  [in6] -> M156/5(EB1)
  [in7] -> M156/6(CT2)
  [in8] -> M156/7(F2)
  [in9] -> M156/8(E2)
  [in11] -> M156/9(T2)
  [in12] -> M156/10(EB2)
  M156/1(LL1) -> Eval155/1(In1)
  M156/2(LL2) -> Eval155/2(In2)
  Eval155/1(Out1) -> To Workspace155/1
  [in1] -> M157/1(CT1)
  [in2] -> M157/2(F1)
  [in3] -> M157/3(E1)
  [in5] -> M157/4(T1)
  [in6] -> M157/5(EB1)
  [in7] -> M157/6(CT2)
  [in8] -> M157/7(F2)
  [in9] -> M157/8(E2)
  [in11] -> M157/9(T2)
  [in12] -> M157/10(EB2)
  M157/1(LL1) -> Eval156/1(In1)
  M157/2(LL2) -> Eval156/2(In2)
  Eval156/1(Out1) -> To Workspace156/1
  [in1] -> M158/1(CT1)
  [in2] -> M158/2(F1)
  [in3] -> M158/3(E1)
  [in5] -> M158/4(T1)
  [in6] -> M158/5(EB1)
  [in7] -> M158/6(CT2)
  [in8] -> M158/7(F2)
  [in9] -> M158/8(E2)
  [in11] -> M158/9(T2)
  [in12] -> M158/10(EB2)
  M158/1(LL1) -> Eval157/1(In1)
  M158/2(LL2) -> Eval157/2(In2)
  Eval157/1(Out1) -> To Workspace157/1
  [in1] -> M159/1(CT1)
  [in2] -> M159/2(F1)
  [in3] -> M159/3(E1)
  [in5] -> M159/4(T1)
  [in6] -> M159/5(EB1)
  [in7] -> M159/6(CT2)
  [in8] -> M159/7(F2)
  [in9] -> M159/8(E2)
  [in11] -> M159/9(T2)
  [in12] -> M159/10(EB2)
  M159/1(LL1) -> Eval158/1(In1)
  M159/2(LL2) -> Eval158/2(In2)
  Eval158/1(Out1) -> To Workspace158/1
  [in1] -> M160/1(CT1)
  [in2] -> M160/2(F1)
  [in3] -> M160/3(E1)
  [in5] -> M160/4(T1)
  [in6] -> M160/5(EB1)
  [in7] -> M160/6(CT2)
  [in8] -> M160/7(F2)
  [in9] -> M160/8(E2)
  [in11] -> M160/9(T2)
  [in12] -> M160/10(EB2)
  M160/1(LL1) -> Eval159/1(In1)
  M160/2(LL2) -> Eval159/2(In2)
  Eval159/1(Out1) -> To Workspace159/1
  [in1] -> M161/1(CT1)
  [in2] -> M161/2(F1)
  [in3] -> M161/3(E1)
  [in5] -> M161/4(T1)
  [in6] -> M161/5(EB1)
  [in7] -> M161/6(CT2)
  [in8] -> M161/7(F2)
  [in9] -> M161/8(E2)
  [in11] -> M161/9(T2)
  [in12] -> M161/10(EB2)
  M161/1(LL1) -> Eval160/1(In1)
  M161/2(LL2) -> Eval160/2(In2)
  Eval160/1(Out1) -> To Workspace160/1
  [in1] -> M162/1(CT1)
  [in2] -> M162/2(F1)
  [in3] -> M162/3(E1)
  [in5] -> M162/4(T1)
  [in6] -> M162/5(EB1)
  [in7] -> M162/6(CT2)
  [in8] -> M162/7(F2)
  [in9] -> M162/8(E2)
  [in11] -> M162/9(T2)
  [in12] -> M162/10(EB2)
  M162/1(LL1) -> Eval161/1(In1)
  M162/2(LL2) -> Eval161/2(In2)
  Eval161/1(Out1) -> To Workspace161/1
  [in1] -> M163/1(CT1)
  [in2] -> M163/2(F1)
  [in3] -> M163/3(E1)
  [in5] -> M163/4(T1)
  [in6] -> M163/5(EB1)
  [in7] -> M163/6(CT2)
  [in8] -> M163/7(F2)
  [in9] -> M163/8(E2)
  [in11] -> M163/9(T2)
  [in12] -> M163/10(EB2)
  M163/1(LL1) -> Eval162/1(In1)
  M163/2(LL2) -> Eval162/2(In2)
  Eval162/1(Out1) -> To Workspace162/1
  [in1] -> M164/1(CT1)
  [in2] -> M164/2(F1)
  [in3] -> M164/3(E1)
  [in5] -> M164/4(T1)
  [in6] -> M164/5(EB1)
  [in7] -> M164/6(CT2)
  [in8] -> M164/7(F2)
  [in9] -> M164/8(E2)
  [in11] -> M164/9(T2)
  [in12] -> M164/10(EB2)
  M164/1(LL1) -> Eval163/1(In1)
  M164/2(LL2) -> Eval163/2(In2)
  Eval163/1(Out1) -> To Workspace163/1
  [in1] -> M226/1(CT1)
  [in2] -> M226/2(F1)
  [in3] -> M226/3(E1)
  [in5] -> M226/4(T1)
  [in6] -> M226/5(EB1)
  [in7] -> M226/6(CT2)
  [in8] -> M226/7(F2)
  [in9] -> M226/8(E2)
  [in11] -> M226/9(T2)
  [in12] -> M226/10(EB2)
  M226/1(LL1) -> Eval225/1(In1)
  M226/2(LL2) -> Eval225/2(In2)
  Eval225/1(Out1) -> To Workspace225/1
  [in1] -> M227/1(CT1)
  [in2] -> M227/2(F1)
  [in3] -> M227/3(E1)
  [in5] -> M227/4(T1)
  [in6] -> M227/5(EB1)
  [in7] -> M227/6(CT2)
  [in8] -> M227/7(F2)
  [in9] -> M227/8(E2)
  [in11] -> M227/9(T2)
  [in12] -> M227/10(EB2)
  M227/1(LL1) -> Eval226/1(In1)
  M227/2(LL2) -> Eval226/2(In2)
  Eval226/1(Out1) -> To Workspace226/1
  [in1] -> M228/1(CT1)
  [in2] -> M228/2(F1)
  [in3] -> M228/3(E1)
  [in5] -> M228/4(T1)
  [in6] -> M228/5(EB1)
  [in7] -> M228/6(CT2)
  [in8] -> M228/7(F2)
  [in9] -> M228/8(E2)
  [in11] -> M228/9(T2)
  [in12] -> M228/10(EB2)
  M228/1(LL1) -> Eval227/1(In1)
  M228/2(LL2) -> Eval227/2(In2)
  Eval227/1(Out1) -> To Workspace227/1
  [in1] -> M229/1(CT1)
  [in2] -> M229/2(F1)
  [in3] -> M229/3(E1)
  [in5] -> M229/4(T1)
  [in6] -> M229/5(EB1)
  [in7] -> M229/6(CT2)
  [in8] -> M229/7(F2)
  [in9] -> M229/8(E2)
  [in11] -> M229/9(T2)
  [in12] -> M229/10(EB2)
  M229/1(LL1) -> Eval228/1(In1)
  M229/2(LL2) -> Eval228/2(In2)
  Eval228/1(Out1) -> To Workspace228/1
  [in1] -> M230/1(CT1)
  [in2] -> M230/2(F1)
  [in3] -> M230/3(E1)
  [in5] -> M230/4(T1)
  [in6] -> M230/5(EB1)
  [in7] -> M230/6(CT2)
  [in8] -> M230/7(F2)
  [in9] -> M230/8(E2)
  [in11] -> M230/9(T2)
  [in12] -> M230/10(EB2)
  M230/1(LL1) -> Eval229/1(In1)
  M230/2(LL2) -> Eval229/2(In2)
  Eval229/1(Out1) -> To Workspace229/1
  Inputs/1(CT1) -> dtc_CT1/1
  dtc_CT1/1 -> CPSUT/1(CT1), [in1]
  Inputs/2(F1) -> dtc_F1/1
  dtc_F1/1 -> CPSUT/2(F1), [in2]
  Inputs/3(E1) -> dtc_E1/1
  dtc_E1/1 -> CPSUT/3(E1), [in3]
  Inputs/4(T1) -> dtc_T1/1
  dtc_T1/1 -> CPSUT/4(T1), [in5]
  Inputs/5(EB1) -> dtc_EB1/1
  dtc_EB1/1 -> CPSUT/5(EB1), [in6]
  Inputs/6(CT2) -> dtc_CT2/1
  dtc_CT2/1 -> CPSUT/6(CT2), [in7]
  Inputs/7(F2) -> dtc_F2/1
  dtc_F2/1 -> CPSUT/7(F2), [in8]
  Inputs/8(E2) -> dtc_E2/1
  dtc_E2/1 -> CPSUT/8(E2), [in9]
  Inputs/9(T2) -> dtc_T2/1
  dtc_T2/1 -> CPSUT/9(T2), [in11]
  Inputs/10(EB2) -> dtc_EB2/1
  dtc_EB2/1 -> CPSUT/10(EB2), [in12]

== system c00012M_harness/CPSUT ==
  note: VALUES
      | ---------------------------------
      | ControlType = 1 | 2 | 3
      | FillTank = 0 | 1
      | EmptyTank = 0 | 1
      | ManualReference between 0 and 1
      | Tempreature between 0 and 100
      | EmergencyButton = 0 | 1
      | LiquidLevel between 0 and 1 (hmax)
  note: Inputs For Tank2
  note: NAMES
      | --------------------------------------------
      | CT1 = ControlType Tank 1
      | F1 = Fill Tank 1
      | E1 = Empty Tank 1
      | MR1 = Manual Reference Tank1
      | T1 = Temperature Tank 1
      | EB1 = Emergency Button Tank 1
      | LL1 = Liquid Level 1
  note: Inputs For Tank3
  note: Inputs For Tank1
  CT1 : Inport
  F1 : Inport  Port=2
  E1 : Inport  Port=3
  T1 : Inport  Port=4
  EB1 : Inport  Port=5
  CT2 : Inport  Port=6
  F2 : Inport  Port=7
  E2 : Inport  Port=8
  T2 : Inport  Port=9
  EB2 : Inport  Port=10
  Tank1 : Subsystem
  Tank2 : Subsystem
  LL1 : Outport
  LL2 : Outport  Port=2
  wires:
  EB1/1 -> Tank1/5(EB1)
  Tank2/1(LL2) -> LL2/1, Tank1/6(LL2)
  EB2/1 -> Tank2/5(EB2)
  CT2/1 -> Tank2/1(CT2)
  T1/1 -> Tank1/4(T1)
  Tank1/1(LL1) -> LL1/1, Tank2/6(LL1)
  F2/1 -> Tank2/2(F2)
  E2/1 -> Tank2/3(E2)
  F1/1 -> Tank1/2(F1)
  E1/1 -> Tank1/3(E1)
  T2/1 -> Tank2/4(T2)
  CT1/1 -> Tank1/1(CT1)

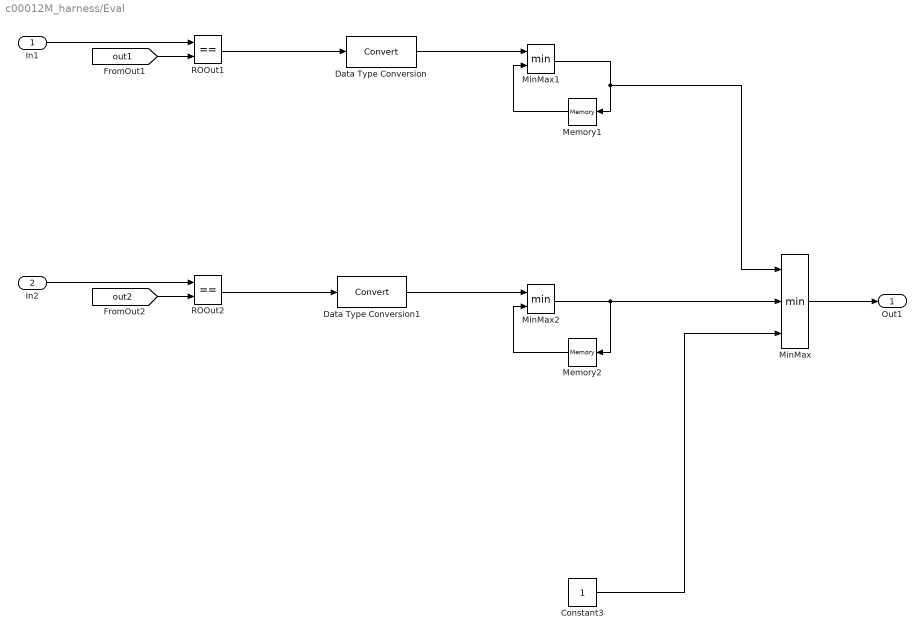
== system c00012M_harness/Eval ==
  In1 : Inport
  In2 : Inport  Port=2
  Constant3 : Constant
  Data Type Conversion : DataTypeConversion
  Data Type Conversion1 : DataTypeConversion
  Memory1 : Memory  InitialCondition=1
  Memory2 : Memory  InitialCondition=1
  MinMax : MinMax  Inputs=3
  MinMax1 : MinMax  Inputs=2
  MinMax2 : MinMax  Inputs=2
  ROOut1 : RelationalOperator  Operator===  OutDataTypeStr=boolean  RndMeth=Simplest
  ROOut2 : RelationalOperator  Operator===  OutDataTypeStr=boolean  RndMeth=Simplest
  Out1 : Outport
  wires:
  MinMax/1 -> Out1/1
  [out1] -> ROOut1/2
  In2/1 -> ROOut2/1
  In1/1 -> ROOut1/1
  [out2] -> ROOut2/2
  Memory1/1 -> MinMax1/2
  ROOut2/1 -> Data Type Conversion1/1
  Memory2/1 -> MinMax2/2
  ROOut1/1 -> Data Type Conversion/1
  MinMax2/1 -> Memory2/1, MinMax/2
  MinMax1/1 -> MinMax/1, Memory1/1
  Data Type Conversion/1 -> MinMax1/1
  Data Type Conversion1/1 -> MinMax2/1
  Constant3/1 -> MinMax/3

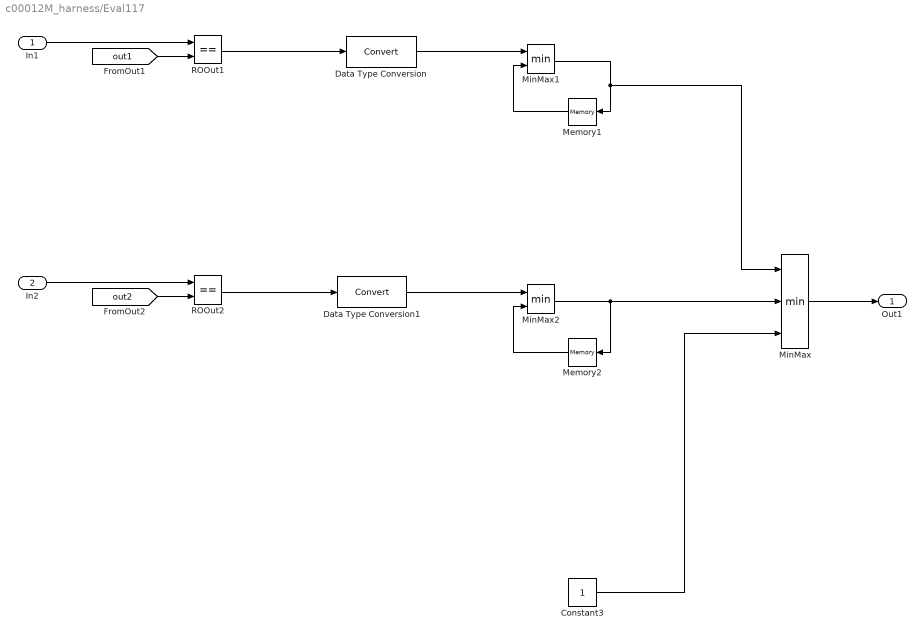
== system c00012M_harness/Eval117 ==
  In1 : Inport
  In2 : Inport  Port=2
  Constant3 : Constant
  Data Type Conversion : DataTypeConversion
  Data Type Conversion1 : DataTypeConversion
  Memory1 : Memory  InitialCondition=1
  Memory2 : Memory  InitialCondition=1
  MinMax : MinMax  Inputs=3
  MinMax1 : MinMax  Inputs=2
  MinMax2 : MinMax  Inputs=2
  ROOut1 : RelationalOperator  Operator===  OutDataTypeStr=boolean  RndMeth=Simplest
  ROOut2 : RelationalOperator  Operator===  OutDataTypeStr=boolean  RndMeth=Simplest
  Out1 : Outport
  wires:
  Data Type Conversion1/1 -> MinMax2/1
  Data Type Conversion/1 -> MinMax1/1
  MinMax1/1 -> Memory1/1, MinMax/1
  MinMax2/1 -> MinMax/2, Memory2/1
  ROOut1/1 -> Data Type Conversion/1
  Memory2/1 -> MinMax2/2
  ROOut2/1 -> Data Type Conversion1/1
  Memory1/1 -> MinMax1/2
  [out2] -> ROOut2/2
  In1/1 -> ROOut1/1
  In2/1 -> ROOut2/1
  [out1] -> ROOut1/2
  MinMax/1 -> Out1/1
  Constant3/1 -> MinMax/3

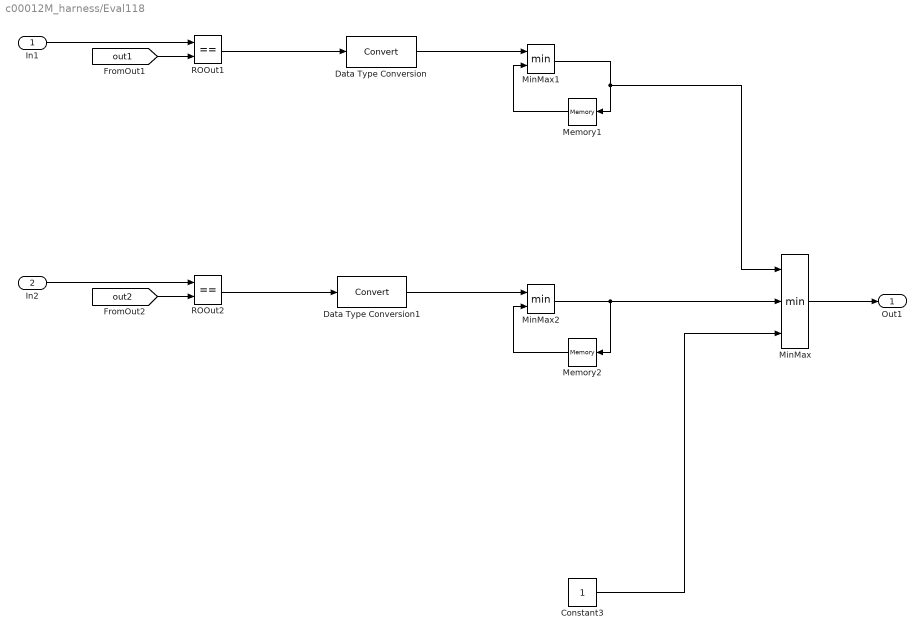
== system c00012M_harness/Eval118 ==
  In1 : Inport
  In2 : Inport  Port=2
  Constant3 : Constant
  Data Type Conversion : DataTypeConversion
  Data Type Conversion1 : DataTypeConversion
  Memory1 : Memory  InitialCondition=1
  Memory2 : Memory  InitialCondition=1
  MinMax : MinMax  Inputs=3
  MinMax1 : MinMax  Inputs=2
  MinMax2 : MinMax  Inputs=2
  ROOut1 : RelationalOperator  Operator===  OutDataTypeStr=boolean  RndMeth=Simplest
  ROOut2 : RelationalOperator  Operator===  OutDataTypeStr=boolean  RndMeth=Simplest
  Out1 : Outport
  wires:
  Data Type Conversion1/1 -> MinMax2/1
  Data Type Conversion/1 -> MinMax1/1
  MinMax1/1 -> Memory1/1, MinMax/1
  MinMax2/1 -> MinMax/2, Memory2/1
  ROOut1/1 -> Data Type Conversion/1
  Memory2/1 -> MinMax2/2
  ROOut2/1 -> Data Type Conversion1/1
  Memory1/1 -> MinMax1/2
  [out2] -> ROOut2/2
  In1/1 -> ROOut1/1
  In2/1 -> ROOut2/1
  [out1] -> ROOut1/2
  MinMax/1 -> Out1/1
  Constant3/1 -> MinMax/3

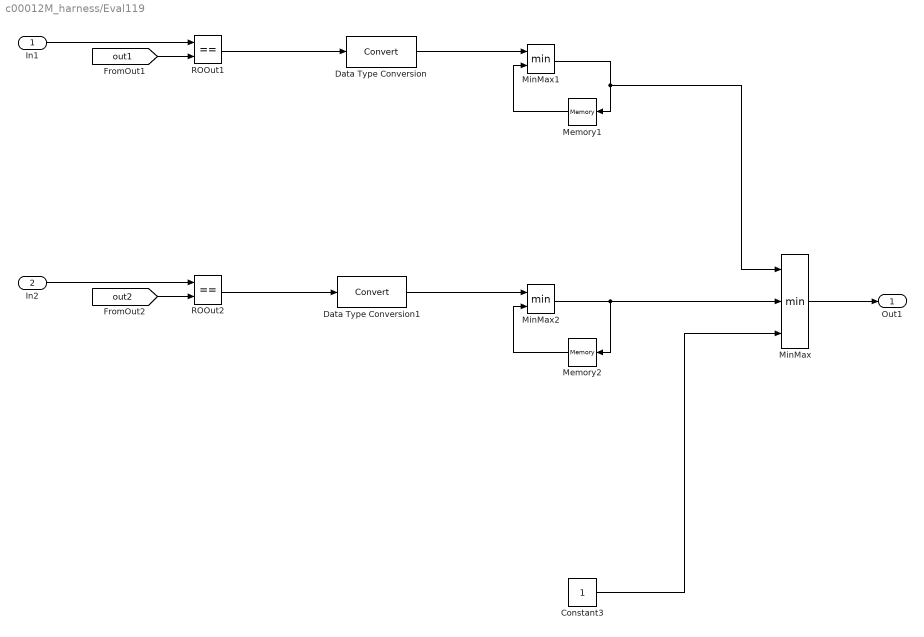
== system c00012M_harness/Eval119 ==
  In1 : Inport
  In2 : Inport  Port=2
  Constant3 : Constant
  Data Type Conversion : DataTypeConversion
  Data Type Conversion1 : DataTypeConversion
  Memory1 : Memory  InitialCondition=1
  Memory2 : Memory  InitialCondition=1
  MinMax : MinMax  Inputs=3
  MinMax1 : MinMax  Inputs=2
  MinMax2 : MinMax  Inputs=2
  ROOut1 : RelationalOperator  Operator===  OutDataTypeStr=boolean  RndMeth=Simplest
  ROOut2 : RelationalOperator  Operator===  OutDataTypeStr=boolean  RndMeth=Simplest
  Out1 : Outport
  wires:
  Data Type Conversion1/1 -> MinMax2/1
  Data Type Conversion/1 -> MinMax1/1
  MinMax1/1 -> Memory1/1, MinMax/1
  MinMax2/1 -> MinMax/2, Memory2/1
  ROOut1/1 -> Data Type Conversion/1
  Memory2/1 -> MinMax2/2
  ROOut2/1 -> Data Type Conversion1/1
  Memory1/1 -> MinMax1/2
  [out2] -> ROOut2/2
  In1/1 -> ROOut1/1
  In2/1 -> ROOut2/1
  [out1] -> ROOut1/2
  MinMax/1 -> Out1/1
  Constant3/1 -> MinMax/3

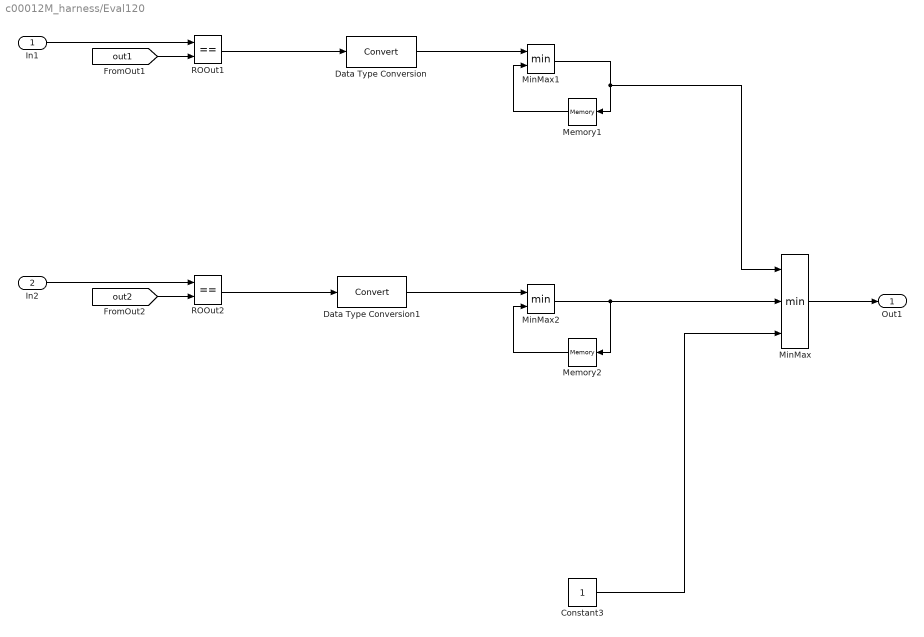
== system c00012M_harness/Eval120 ==
  In1 : Inport
  In2 : Inport  Port=2
  Constant3 : Constant
  Data Type Conversion : DataTypeConversion
  Data Type Conversion1 : DataTypeConversion
  Memory1 : Memory  InitialCondition=1
  Memory2 : Memory  InitialCondition=1
  MinMax : MinMax  Inputs=3
  MinMax1 : MinMax  Inputs=2
  MinMax2 : MinMax  Inputs=2
  ROOut1 : RelationalOperator  Operator===  OutDataTypeStr=boolean  RndMeth=Simplest
  ROOut2 : RelationalOperator  Operator===  OutDataTypeStr=boolean  RndMeth=Simplest
  Out1 : Outport
  wires:
  Data Type Conversion1/1 -> MinMax2/1
  Data Type Conversion/1 -> MinMax1/1
  MinMax1/1 -> Memory1/1, MinMax/1
  MinMax2/1 -> MinMax/2, Memory2/1
  ROOut1/1 -> Data Type Conversion/1
  Memory2/1 -> MinMax2/2
  ROOut2/1 -> Data Type Conversion1/1
  Memory1/1 -> MinMax1/2
  [out2] -> ROOut2/2
  In1/1 -> ROOut1/1
  In2/1 -> ROOut2/1
  [out1] -> ROOut1/2
  MinMax/1 -> Out1/1
  Constant3/1 -> MinMax/3

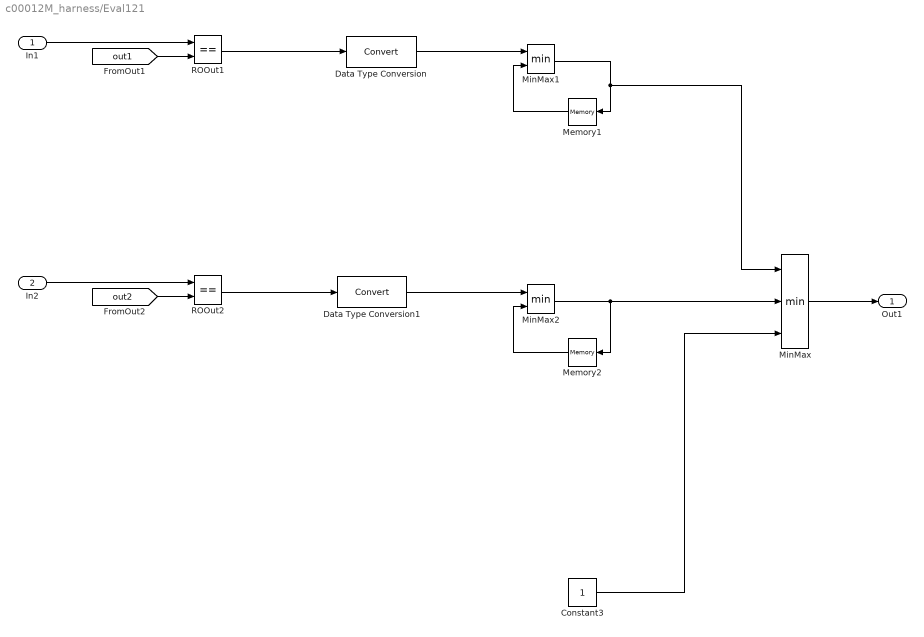
== system c00012M_harness/Eval121 ==
  In1 : Inport
  In2 : Inport  Port=2
  Constant3 : Constant
  Data Type Conversion : DataTypeConversion
  Data Type Conversion1 : DataTypeConversion
  Memory1 : Memory  InitialCondition=1
  Memory2 : Memory  InitialCondition=1
  MinMax : MinMax  Inputs=3
  MinMax1 : MinMax  Inputs=2
  MinMax2 : MinMax  Inputs=2
  ROOut1 : RelationalOperator  Operator===  OutDataTypeStr=boolean  RndMeth=Simplest
  ROOut2 : RelationalOperator  Operator===  OutDataTypeStr=boolean  RndMeth=Simplest
  Out1 : Outport
  wires:
  Data Type Conversion1/1 -> MinMax2/1
  Data Type Conversion/1 -> MinMax1/1
  MinMax1/1 -> Memory1/1, MinMax/1
  MinMax2/1 -> MinMax/2, Memory2/1
  ROOut1/1 -> Data Type Conversion/1
  Memory2/1 -> MinMax2/2
  ROOut2/1 -> Data Type Conversion1/1
  Memory1/1 -> MinMax1/2
  [out2] -> ROOut2/2
  In1/1 -> ROOut1/1
  In2/1 -> ROOut2/1
  [out1] -> ROOut1/2
  MinMax/1 -> Out1/1
  Constant3/1 -> MinMax/3

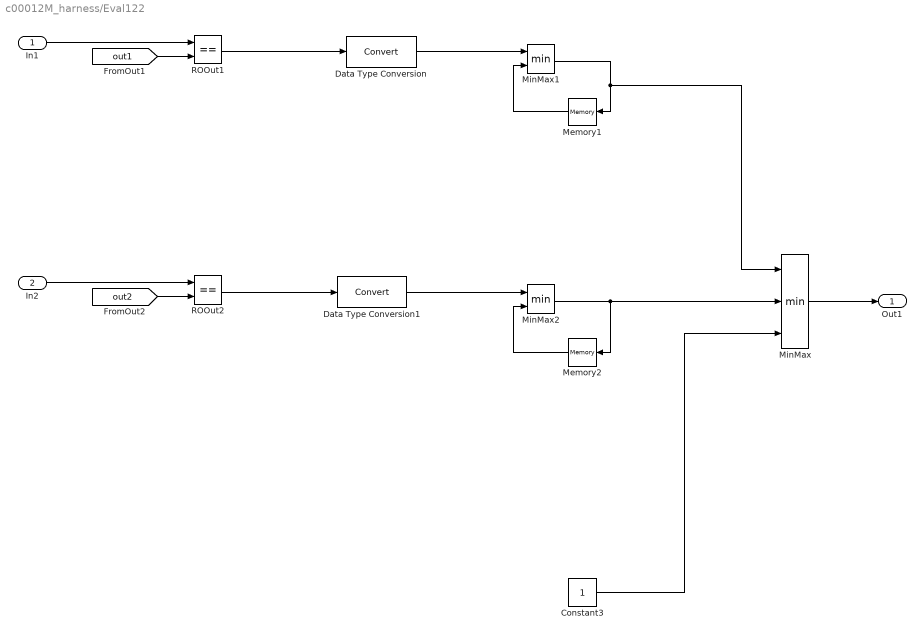
== system c00012M_harness/Eval122 ==
  In1 : Inport
  In2 : Inport  Port=2
  Constant3 : Constant
  Data Type Conversion : DataTypeConversion
  Data Type Conversion1 : DataTypeConversion
  Memory1 : Memory  InitialCondition=1
  Memory2 : Memory  InitialCondition=1
  MinMax : MinMax  Inputs=3
  MinMax1 : MinMax  Inputs=2
  MinMax2 : MinMax  Inputs=2
  ROOut1 : RelationalOperator  Operator===  OutDataTypeStr=boolean  RndMeth=Simplest
  ROOut2 : RelationalOperator  Operator===  OutDataTypeStr=boolean  RndMeth=Simplest
  Out1 : Outport
  wires:
  Data Type Conversion1/1 -> MinMax2/1
  Data Type Conversion/1 -> MinMax1/1
  MinMax1/1 -> Memory1/1, MinMax/1
  MinMax2/1 -> MinMax/2, Memory2/1
  ROOut1/1 -> Data Type Conversion/1
  Memory2/1 -> MinMax2/2
  ROOut2/1 -> Data Type Conversion1/1
  Memory1/1 -> MinMax1/2
  [out2] -> ROOut2/2
  In1/1 -> ROOut1/1
  In2/1 -> ROOut2/1
  [out1] -> ROOut1/2
  MinMax/1 -> Out1/1
  Constant3/1 -> MinMax/3

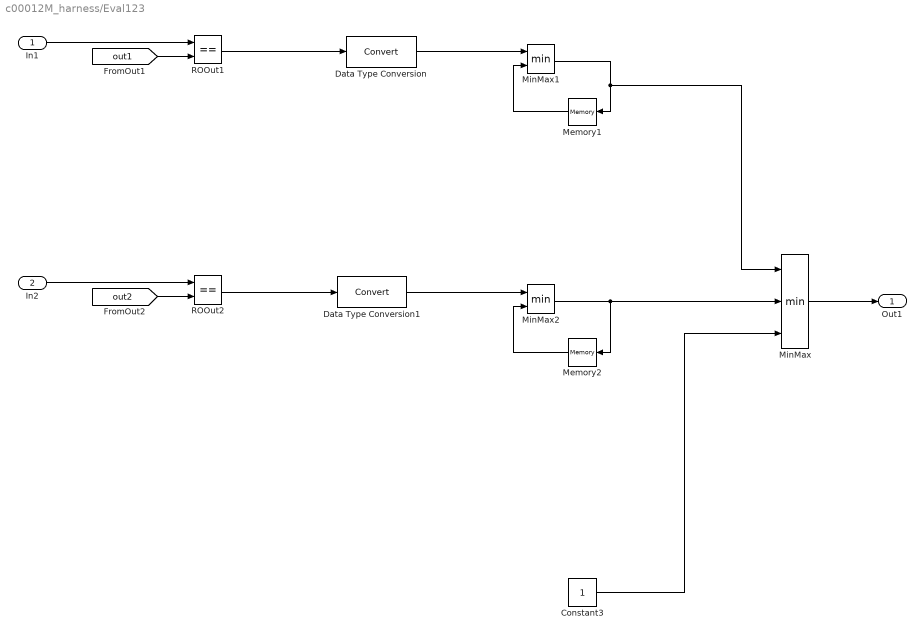
== system c00012M_harness/Eval123 ==
  In1 : Inport
  In2 : Inport  Port=2
  Constant3 : Constant
  Data Type Conversion : DataTypeConversion
  Data Type Conversion1 : DataTypeConversion
  Memory1 : Memory  InitialCondition=1
  Memory2 : Memory  InitialCondition=1
  MinMax : MinMax  Inputs=3
  MinMax1 : MinMax  Inputs=2
  MinMax2 : MinMax  Inputs=2
  ROOut1 : RelationalOperator  Operator===  OutDataTypeStr=boolean  RndMeth=Simplest
  ROOut2 : RelationalOperator  Operator===  OutDataTypeStr=boolean  RndMeth=Simplest
  Out1 : Outport
  wires:
  Data Type Conversion1/1 -> MinMax2/1
  Data Type Conversion/1 -> MinMax1/1
  MinMax1/1 -> Memory1/1, MinMax/1
  MinMax2/1 -> MinMax/2, Memory2/1
  ROOut1/1 -> Data Type Conversion/1
  Memory2/1 -> MinMax2/2
  ROOut2/1 -> Data Type Conversion1/1
  Memory1/1 -> MinMax1/2
  [out2] -> ROOut2/2
  In1/1 -> ROOut1/1
  In2/1 -> ROOut2/1
  [out1] -> ROOut1/2
  MinMax/1 -> Out1/1
  Constant3/1 -> MinMax/3

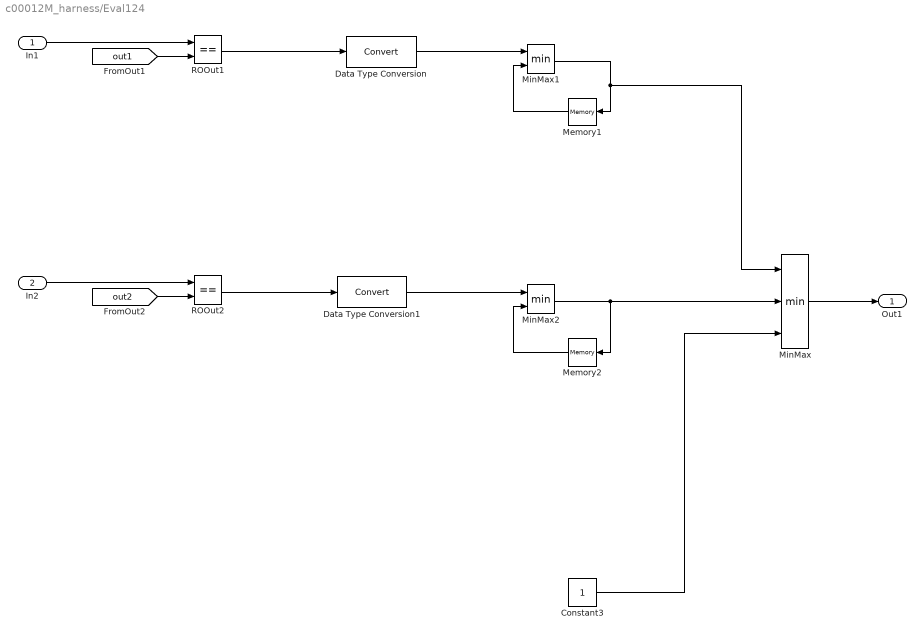
== system c00012M_harness/Eval124 ==
  In1 : Inport
  In2 : Inport  Port=2
  Constant3 : Constant
  Data Type Conversion : DataTypeConversion
  Data Type Conversion1 : DataTypeConversion
  Memory1 : Memory  InitialCondition=1
  Memory2 : Memory  InitialCondition=1
  MinMax : MinMax  Inputs=3
  MinMax1 : MinMax  Inputs=2
  MinMax2 : MinMax  Inputs=2
  ROOut1 : RelationalOperator  Operator===  OutDataTypeStr=boolean  RndMeth=Simplest
  ROOut2 : RelationalOperator  Operator===  OutDataTypeStr=boolean  RndMeth=Simplest
  Out1 : Outport
  wires:
  Data Type Conversion1/1 -> MinMax2/1
  Data Type Conversion/1 -> MinMax1/1
  MinMax1/1 -> Memory1/1, MinMax/1
  MinMax2/1 -> MinMax/2, Memory2/1
  ROOut1/1 -> Data Type Conversion/1
  Memory2/1 -> MinMax2/2
  ROOut2/1 -> Data Type Conversion1/1
  Memory1/1 -> MinMax1/2
  [out2] -> ROOut2/2
  In1/1 -> ROOut1/1
  In2/1 -> ROOut2/1
  [out1] -> ROOut1/2
  MinMax/1 -> Out1/1
  Constant3/1 -> MinMax/3

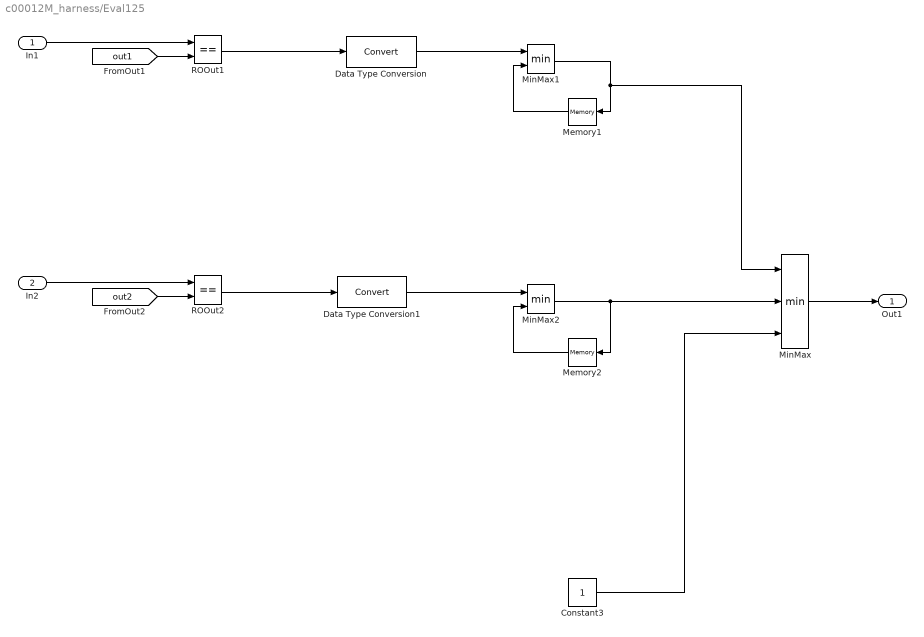
== system c00012M_harness/Eval125 ==
  In1 : Inport
  In2 : Inport  Port=2
  Constant3 : Constant
  Data Type Conversion : DataTypeConversion
  Data Type Conversion1 : DataTypeConversion
  Memory1 : Memory  InitialCondition=1
  Memory2 : Memory  InitialCondition=1
  MinMax : MinMax  Inputs=3
  MinMax1 : MinMax  Inputs=2
  MinMax2 : MinMax  Inputs=2
  ROOut1 : RelationalOperator  Operator===  OutDataTypeStr=boolean  RndMeth=Simplest
  ROOut2 : RelationalOperator  Operator===  OutDataTypeStr=boolean  RndMeth=Simplest
  Out1 : Outport
  wires:
  Data Type Conversion1/1 -> MinMax2/1
  Data Type Conversion/1 -> MinMax1/1
  MinMax1/1 -> Memory1/1, MinMax/1
  MinMax2/1 -> MinMax/2, Memory2/1
  ROOut1/1 -> Data Type Conversion/1
  Memory2/1 -> MinMax2/2
  ROOut2/1 -> Data Type Conversion1/1
  Memory1/1 -> MinMax1/2
  [out2] -> ROOut2/2
  In1/1 -> ROOut1/1
  In2/1 -> ROOut2/1
  [out1] -> ROOut1/2
  MinMax/1 -> Out1/1
  Constant3/1 -> MinMax/3

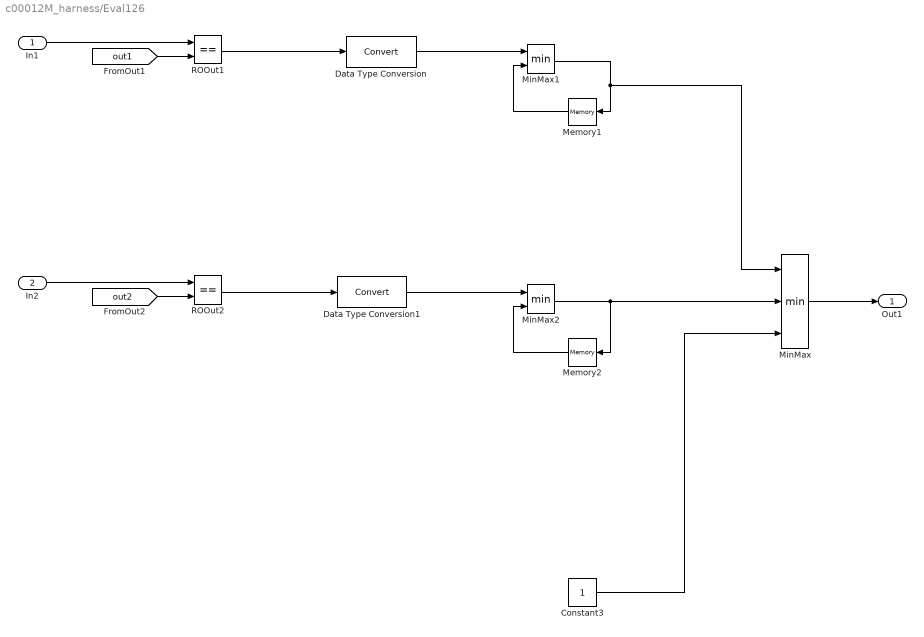
== system c00012M_harness/Eval126 ==
  In1 : Inport
  In2 : Inport  Port=2
  Constant3 : Constant
  Data Type Conversion : DataTypeConversion
  Data Type Conversion1 : DataTypeConversion
  Memory1 : Memory  InitialCondition=1
  Memory2 : Memory  InitialCondition=1
  MinMax : MinMax  Inputs=3
  MinMax1 : MinMax  Inputs=2
  MinMax2 : MinMax  Inputs=2
  ROOut1 : RelationalOperator  Operator===  OutDataTypeStr=boolean  RndMeth=Simplest
  ROOut2 : RelationalOperator  Operator===  OutDataTypeStr=boolean  RndMeth=Simplest
  Out1 : Outport
  wires:
  Data Type Conversion1/1 -> MinMax2/1
  Data Type Conversion/1 -> MinMax1/1
  MinMax1/1 -> Memory1/1, MinMax/1
  MinMax2/1 -> MinMax/2, Memory2/1
  ROOut1/1 -> Data Type Conversion/1
  Memory2/1 -> MinMax2/2
  ROOut2/1 -> Data Type Conversion1/1
  Memory1/1 -> MinMax1/2
  [out2] -> ROOut2/2
  In1/1 -> ROOut1/1
  In2/1 -> ROOut2/1
  [out1] -> ROOut1/2
  MinMax/1 -> Out1/1
  Constant3/1 -> MinMax/3

== system c00012M_harness/Eval139 ==
  In1 : Inport
  In2 : Inport  Port=2
  Constant3 : Constant
  Data Type Conversion : DataTypeConversion
  Data Type Conversion1 : DataTypeConversion
  Memory1 : Memory  InitialCondition=1
  Memory2 : Memory  InitialCondition=1
  MinMax : MinMax  Inputs=3
  MinMax1 : MinMax  Inputs=2
  MinMax2 : MinMax  Inputs=2
  ROOut1 : RelationalOperator  Operator===  OutDataTypeStr=boolean  RndMeth=Simplest
  ROOut2 : RelationalOperator  Operator===  OutDataTypeStr=boolean  RndMeth=Simplest
  Out1 : Outport
  wires:
  Data Type Conversion1/1 -> MinMax2/1
  Data Type Conversion/1 -> MinMax1/1
  MinMax1/1 -> Memory1/1, MinMax/1
  MinMax2/1 -> MinMax/2, Memory2/1
  ROOut1/1 -> Data Type Conversion/1
  Memory2/1 -> MinMax2/2
  ROOut2/1 -> Data Type Conversion1/1
  Memory1/1 -> MinMax1/2
  [out2] -> ROOut2/2
  In1/1 -> ROOut1/1
  In2/1 -> ROOut2/1
  [out1] -> ROOut1/2
  MinMax/1 -> Out1/1
  Constant3/1 -> MinMax/3

== system c00012M_harness/Eval140 ==
  In1 : Inport
  In2 : Inport  Port=2
  Constant3 : Constant
  Data Type Conversion : DataTypeConversion
  Data Type Conversion1 : DataTypeConversion
  Memory1 : Memory  InitialCondition=1
  Memory2 : Memory  InitialCondition=1
  MinMax : MinMax  Inputs=3
  MinMax1 : MinMax  Inputs=2
  MinMax2 : MinMax  Inputs=2
  ROOut1 : RelationalOperator  Operator===  OutDataTypeStr=boolean  RndMeth=Simplest
  ROOut2 : RelationalOperator  Operator===  OutDataTypeStr=boolean  RndMeth=Simplest
  Out1 : Outport
  wires:
  Data Type Conversion1/1 -> MinMax2/1
  Data Type Conversion/1 -> MinMax1/1
  MinMax1/1 -> Memory1/1, MinMax/1
  MinMax2/1 -> MinMax/2, Memory2/1
  ROOut1/1 -> Data Type Conversion/1
  Memory2/1 -> MinMax2/2
  ROOut2/1 -> Data Type Conversion1/1
  Memory1/1 -> MinMax1/2
  [out2] -> ROOut2/2
  In1/1 -> ROOut1/1
  In2/1 -> ROOut2/1
  [out1] -> ROOut1/2
  MinMax/1 -> Out1/1
  Constant3/1 -> MinMax/3
